simulink model "yek_alef_tanaka"  (R2024a)
settings: Solver=ode15s  StartTime=0.0  StopTime=9000  RelTol=1e-3
settings Model: Creator=MAHDI  LastModifiedBy=ASUS
settings DebuggingCC: UnconnectedInputMsg=warning  UnconnectedOutputMsg=warning  UnconnectedLineMsg=warning
settings ModelReferenceCC: EnableRefExpFcnMdlSchedulingChecks=on
settings RTWCC: GPUComputeCapability=3.5  DLArmComputeVersion=19.05

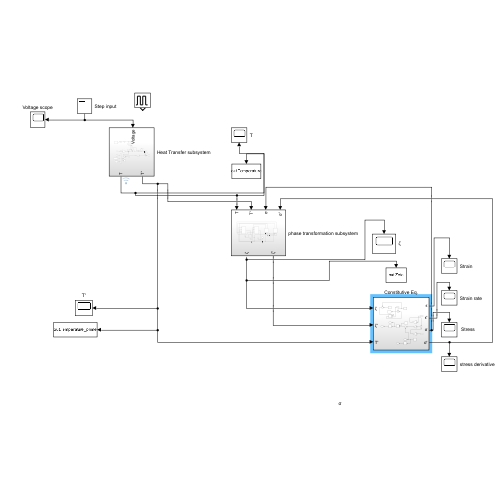
[thumbnail: Simulink's stored preview of the top-level diagram]
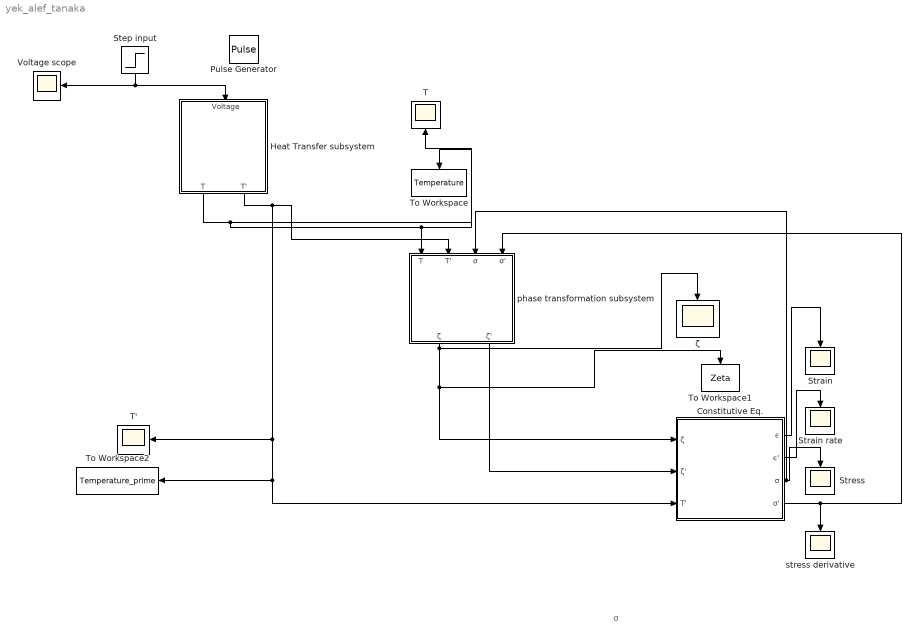
== system yek_alef_tanaka ==
  note: σ
  " Stress" : Scope
  Constitutive Eq. : Subsystem
  Heat Transfer subsystem : Subsystem
  Pulse Generator : DiscretePulseGenerator  PulseType=Time based  Period=100  PulseWidth=5
  Step input : Step  Time=70  Before=1  After=0  SampleTime=0
  Strain : Scope
  Strain rate : Scope
  T : Scope
  T' : Scope
  To Workspace : ToWorkspace  VariableName=Temperature  SampleTime=1
  To Workspace1 : ToWorkspace  VariableName=Zeta  SampleTime=1
  To Workspace2 : ToWorkspace  VariableName=Temperature_prime  SampleTime=1
  Voltage scope : Scope
  phase transformation subsystem : Subsystem
  stress derivative : Scope
  ζ : Scope
  wires:
  Constitutive Eq./3(σ) -> phase transformation subsystem/3(σ), " Stress"/1
  Step input/1 -> Voltage scope/1, Heat Transfer subsystem/1(Voltage)
  Heat Transfer subsystem/2(T') -> To Workspace2/1, Constitutive Eq./3(T'), T'/1, phase transformation subsystem/2(T')
  Heat Transfer subsystem/1(T) -> T/1, phase transformation subsystem/1(T), To Workspace/1
  phase transformation subsystem/2(ζ') -> Constitutive Eq./2(ζ')
  Constitutive Eq./1(ϵ) -> Strain/1
  phase transformation subsystem/1(ζ) -> Constitutive Eq./1(ζ), To Workspace1/1, ζ/1
  Constitutive Eq./2(ϵ') -> Strain rate/1
  Constitutive Eq./4(σ') -> phase transformation subsystem/4("σ' "), stress derivative/1

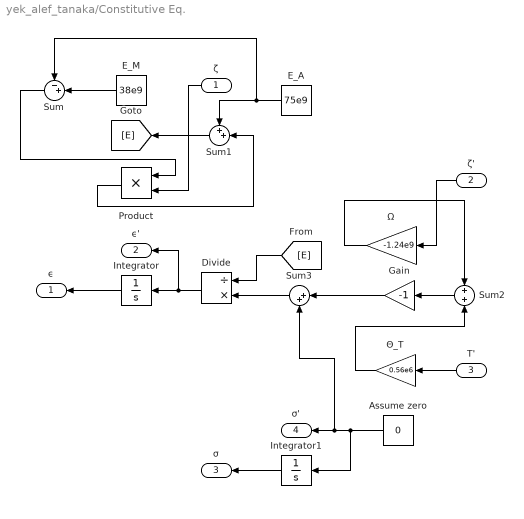
== system yek_alef_tanaka/Constitutive Eq. ==
  ζ : Inport
  ζ' : Inport  Port=2
  T' : Inport  Port=3
  Assume zero : Constant  Value=0
  Divide : Product  Inputs=/*
  E_A : Constant  Value=75e9
  E_M : Constant  Value=38e9
  Gain : Gain  Gain=-1
  Integrator : Integrator
  Integrator1 : Integrator
  Product : Product
  Sum : Sum  Inputs=-+|
  Sum1 : Sum  Inputs=++|
  Sum2 : Sum  Inputs=+|+
  Sum3 : Sum  Inputs=|++
  Θ_T : Gain  Gain=0.56e6
  Ω : Gain  Gain=-1.24e9
  ϵ : Outport
  ϵ' : Outport  Port=2
  σ : Outport  Port=3
  σ' : Outport  Port=4
  wires:
  Sum3/1 -> Divide/2
  Product/1 -> Sum1/2
  Sum1/1 -> [E]
  Sum2/1 -> Gain/1
  Integrator1/1 -> σ/1
  Sum/1 -> Product/1
  E_M/1 -> Sum/2
  E_A/1 -> Sum1/1, Sum/1
  Integrator/1 -> ϵ/1
  Divide/1 -> ϵ'/1, Integrator/1
  ζ/1 -> Product/2
  [E] -> Divide/1
  Ω/1 -> Sum2/1
  Gain/1 -> Sum3/1
  Θ_T/1 -> Sum2/2
  Assume zero/1 -> Sum3/2, σ'/1, Integrator1/1
  ζ'/1 -> Ω/1
  T'/1 -> Θ_T/1

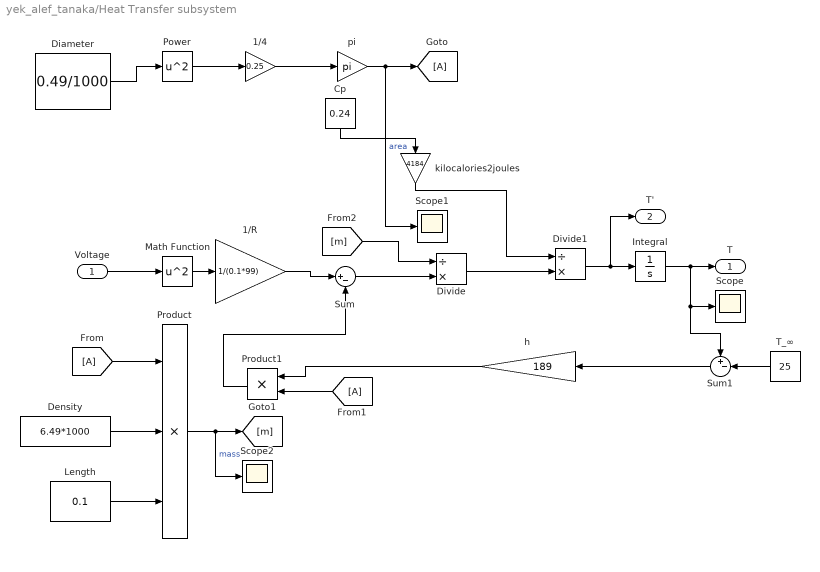
== system yek_alef_tanaka/Heat Transfer subsystem ==
  Voltage : Inport
  1/4 : Gain  Gain=0.25
  1/R : Gain  Gain=1/(0.1*99)
  Cp : Constant  Value=0.24
  Density : Constant  Value=6.49*1000
  Diameter : Constant  Value=0.49/1000
  Divide : Product  Inputs=/*
  Divide1 : Product  Inputs=/*
  From : From
  From1 : From
  Goto : Goto
  Integral : Integrator  InitialCondition=25
  Length : Constant  Value=0.1
  Math Function : Math  Operator=square
  Power : Math  Operator=square
  Product : Product  Inputs=3
  Product1 : Product
  Scope : Scope
  Scope1 : Scope
  Scope2 : Scope
  Sum : Sum  Inputs=|+-
  Sum1 : Sum  Inputs=+-|
  T_∞ : Constant  Value=25
  h : Gain  Gain=189
  "kilocalories2joules " : Gain  Gain=4184
  pi : Gain  Gain=pi
  T : Outport
  T' : Outport  Port=2
  wires:
  Voltage/1 -> Math Function/1
  Diameter/1 -> Power/1
  Density/1 -> Product/2
  From/1 -> Product/1
  1/4/1 -> pi/1
  Length/1 -> Product/3
  Product/1 -> [m], Scope2/1  "mass"
  Power/1 -> 1/4/1
  Math Function/1 -> 1/R/1
  Product1/1 -> Sum/2
  1/R/1 -> Sum/1
  Cp/1 -> "kilocalories2joules "/1
  From1/1 -> Product1/2
  pi/1 -> Scope1/1, Goto/1  "area"
  [m] -> Divide/1
  Sum/1 -> Divide/2
  "kilocalories2joules "/1 -> Divide1/1
  Divide/1 -> Divide1/2
  h/1 -> Product1/1
  Divide1/1 -> Integral/1, T'/1
  Integral/1 -> Sum1/1, Scope/1, T/1
  Sum1/1 -> h/1
  T_∞/1 -> Sum1/2

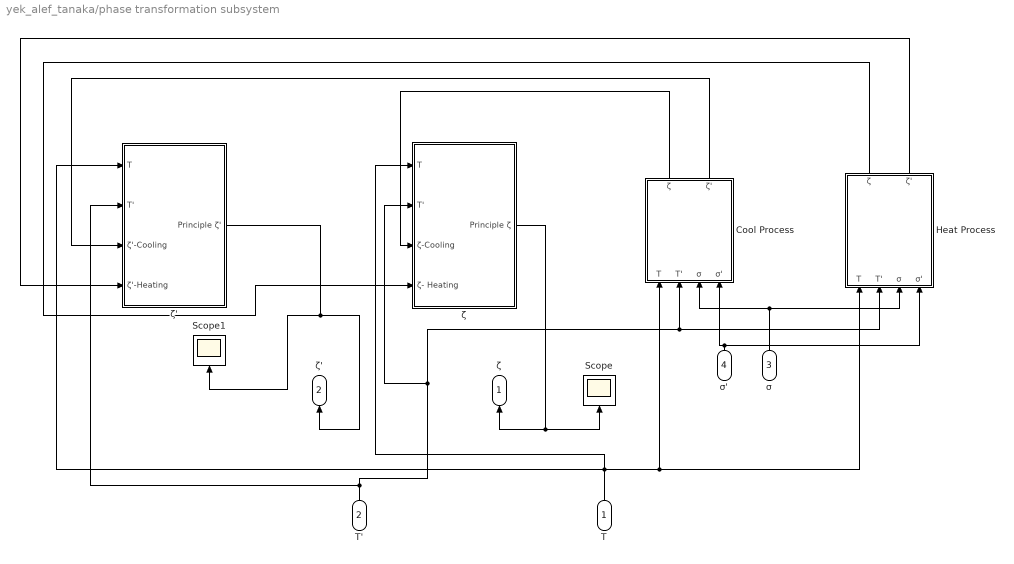
== system yek_alef_tanaka/phase transformation subsystem ==
  T : Inport
  T' : Inport  Port=2
  σ : Inport  Port=3
  "σ' " : Inport  Port=4
  " ζ" : Subsystem
  " ζ'" : Subsystem
  Cool Process : Subsystem
  Heat Process : Subsystem
  Scope : Scope
  Scope1 : Scope
  ζ : Outport
  ζ' : Outport  Port=2
  wires:
  " ζ'"/1(Principle ζ') -> ζ'/1, Scope1/1
  Heat Process/2(ζ') -> " ζ'"/4(ζ'-Heating)
  "σ' "/1 -> Heat Process/4("σ' "), Cool Process/4("σ' ")
  Heat Process/1(ζ) -> " ζ"/4(ζ- Heating)
  Cool Process/2(ζ') -> " ζ'"/3(ζ'-Cooling)
  Cool Process/1(ζ) -> " ζ"/3(ζ-Cooling)
  " ζ"/1(Principle ζ) -> ζ/1, Scope/1
  σ/1 -> Heat Process/3(σ), Cool Process/3(σ)
  T/1 -> " ζ"/1(T), Cool Process/1(T), Heat Process/1(T), " ζ'"/1(T)
  T'/1 -> Cool Process/2(T'), Heat Process/2(T'), " ζ"/2(T'), " ζ'"/2(T')

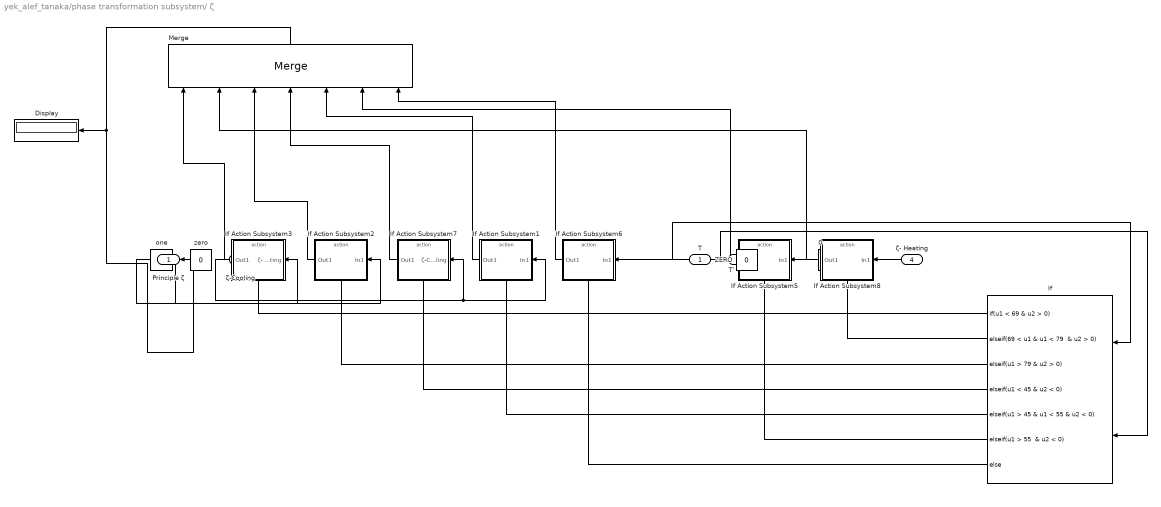
== system yek_alef_tanaka/phase transformation subsystem/ ζ ==
  T : Inport
  T' : Inport  Port=2
  ζ-Cooling : Inport  Port=3
  ζ- Heating : Inport  Port=4
  0 : Constant  Value=0
  Display : Display
  If : If  NumInputs=2  IfExpression=u1 < 69 & u2 > 0  ElseIfExpressions="69 < u1 & u1 < 79  & u2 > 0 , u1 > 79 & u2 > 0 , u1 < 45 & u2 < 0 , u1 > 45 & u1 < 55 & u2 < 0 , u1 > 55  & u2 < 0"
  If Action Subsystem1 : Subsystem  TreatAsAtomicUnit=on
  If Action Subsystem2 : Subsystem  TreatAsAtomicUnit=on
  If Action Subsystem3 : Subsystem  TreatAsAtomicUnit=on
  If Action Subsystem5 : Subsystem  TreatAsAtomicUnit=on
  If Action Subsystem6 : Subsystem  TreatAsAtomicUnit=on
  If Action Subsystem7 : Subsystem  TreatAsAtomicUnit=on
  If Action Subsystem8 : Subsystem  TreatAsAtomicUnit=on
  Merge : Merge  Inputs=7
  ZERO : Constant  Value=0
  one : Constant
  zero : Constant  Value=0
  Principle ζ : Outport
  wires:
  ζ-Cooling/1 -> If Action Subsystem7/1(ζ-Cooling), If Action Subsystem1/1(In1)
  T/1 -> If/1
  T'/1 -> If/2
  one/1 -> If Action Subsystem3/1(ζ- Heating)
  If/1 -> If Action Subsystem3/Action
  zero/1 -> If Action Subsystem2/1(In1)
  If/2 -> If Action Subsystem8/Action
  If/3 -> If Action Subsystem2/Action
  If/4 -> If Action Subsystem7/Action
  If/5 -> If Action Subsystem1/Action
  If/6 -> If Action Subsystem5/Action
  If Action Subsystem8/1(Out1) -> Merge/2
  If/7 -> If Action Subsystem6/Action
  ZERO/1 -> If Action Subsystem6/1(In1)
  0/1 -> If Action Subsystem5/1(In1)
  ζ- Heating/1 -> If Action Subsystem8/1(In1)
  If Action Subsystem3/1(Out1) -> Merge/1
  If Action Subsystem2/1(Out1) -> Merge/3
  If Action Subsystem7/1(Out1) -> Merge/4
  If Action Subsystem1/1(Out1) -> Merge/5
  If Action Subsystem6/1(Out1) -> Merge/7
  If Action Subsystem5/1(Out1) -> Merge/6
  Merge/1 -> Principle ζ/1, Display/1

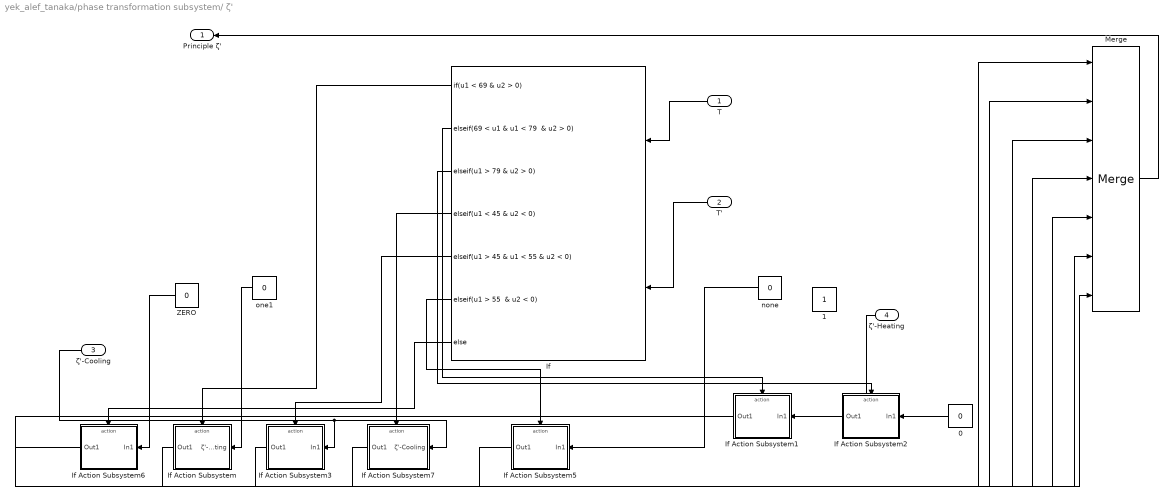
== system yek_alef_tanaka/phase transformation subsystem/ ζ' ==
  T : Inport
  T' : Inport  Port=2
  ζ'-Cooling : Inport  Port=3
  ζ'-Heating : Inport  Port=4
  0 : Constant  Value=0
  1 : Constant
  If : If  NumInputs=2  IfExpression=u1 < 69 & u2 > 0  ElseIfExpressions="69 < u1 & u1 < 79  & u2 > 0 , u1 > 79 & u2 > 0 , u1 < 45 & u2 < 0 , u1 > 45 & u1 < 55 & u2 < 0 , u1 > 55  & u2 < 0"
  If Action Subsystem : Subsystem  TreatAsAtomicUnit=on
  If Action Subsystem1 : Subsystem  TreatAsAtomicUnit=on
  If Action Subsystem2 : Subsystem  TreatAsAtomicUnit=on
  If Action Subsystem3 : Subsystem  TreatAsAtomicUnit=on
  If Action Subsystem5 : Subsystem  TreatAsAtomicUnit=on
  If Action Subsystem6 : Subsystem  TreatAsAtomicUnit=on
  If Action Subsystem7 : Subsystem  TreatAsAtomicUnit=on
  Merge : Merge  Inputs=7
  ZERO : Constant  Value=0
  none : Constant  Value=0
  one1 : Constant  Value=0
  Principle ζ' : Outport
  wires:
  If/5 -> If Action Subsystem3/Action
  ζ'-Heating/1 -> If Action Subsystem1/1(In1)
  If Action Subsystem1/1(Out1) -> Merge/2
  T'/1 -> If/2
  If Action Subsystem7/1(Out1) -> Merge/4
  If/7 -> If Action Subsystem6/Action
  0/1 -> If Action Subsystem2/1(In1)
  If Action Subsystem5/1(Out1) -> Merge/6
  T/1 -> If/1
  If/6 -> If Action Subsystem5/Action
  none/1 -> If Action Subsystem5/1(In1)
  If/4 -> If Action Subsystem7/Action
  If/3 -> If Action Subsystem2/Action
  If/2 -> If Action Subsystem1/Action
  If/1 -> If Action Subsystem/Action
  ζ'-Cooling/1 -> If Action Subsystem7/1(ζ'-Cooling), If Action Subsystem3/1(In1)
  one1/1 -> If Action Subsystem/1(ζ'-Heating)
  ZERO/1 -> If Action Subsystem6/1(In1)
  If Action Subsystem2/1(Out1) -> Merge/3
  If Action Subsystem3/1(Out1) -> Merge/5
  If Action Subsystem/1(Out1) -> Merge/1
  If Action Subsystem6/1(Out1) -> Merge/7
  Merge/1 -> Principle ζ'/1

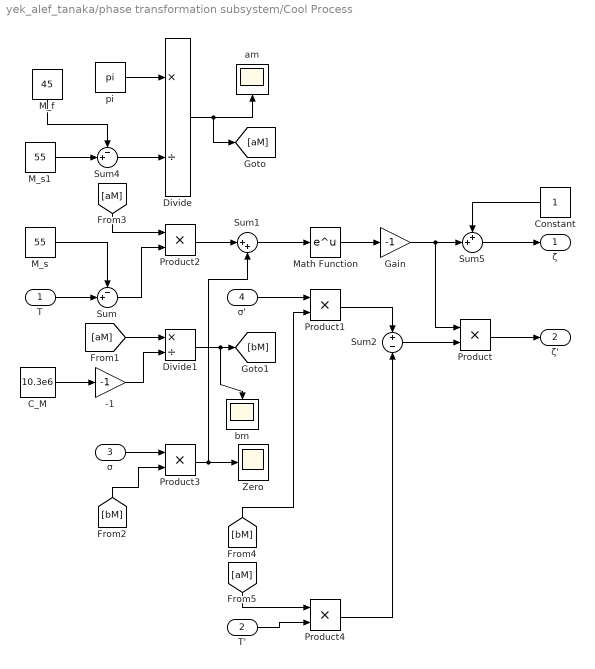
== system yek_alef_tanaka/phase transformation subsystem/Cool Process ==
  T : Inport
  T' : Inport  Port=2
  σ : Inport  Port=3
  "σ' " : Inport  Port=4
  -1 : Gain  Gain=-1
  C_M : Constant  Value=10.3e6
  Constant : Constant
  Divide : Product  Inputs=*/
  Divide1 : Product  Inputs=*/
  Gain : Gain  Gain=-1
  M_f : Constant  Value=45
  M_s : Constant  Value=55
  M_s1 : Constant  Value=55
  Math Function : Math
  Product{,1..4} (5 alike) : Product
  Sum : Sum  Inputs=-+|
  Sum1 : Sum  Inputs=|++
  Sum2 : Sum  Inputs=+|-
  Sum4 : Sum  Inputs=-+|
  Sum5 : Sum  Inputs=++|
  Zero : Scope
  am : Scope
  bm : Scope
  pi : Constant  Value=pi
  ζ : Outport
  ζ' : Outport  Port=2
  wires:
  T/1 -> Sum/2
  M_s1/1 -> Sum4/2
  M_f/1 -> Sum4/1
  M_s/1 -> Sum/1
  Product/1 -> ζ'/1
  Sum4/1 -> Divide/2
  [aM] -> Product4/1
  Product3/1 -> Sum1/2, Zero/1
  pi/1 -> Divide/1
  Product2/1 -> Sum1/1
  [aM] -> Product2/1
  Sum1/1 -> Math Function/1
  C_M/1 -> -1/1
  Sum/1 -> Product2/2
  Sum5/1 -> ζ/1
  Product1/1 -> Sum2/1
  [aM] -> Divide1/1
  -1/1 -> Divide1/2
  σ/1 -> Product3/1
  [bM] -> Product3/2
  Divide/1 -> am/1, [aM]
  Divide1/1 -> bm/1, [bM]
  "σ' "/1 -> Product1/1
  [bM] -> Product1/2
  Gain/1 -> Product/1, Sum5/2
  T'/1 -> Product4/2
  Sum2/1 -> Product/2
  Math Function/1 -> Gain/1
  Product4/1 -> Sum2/2
  Constant/1 -> Sum5/1

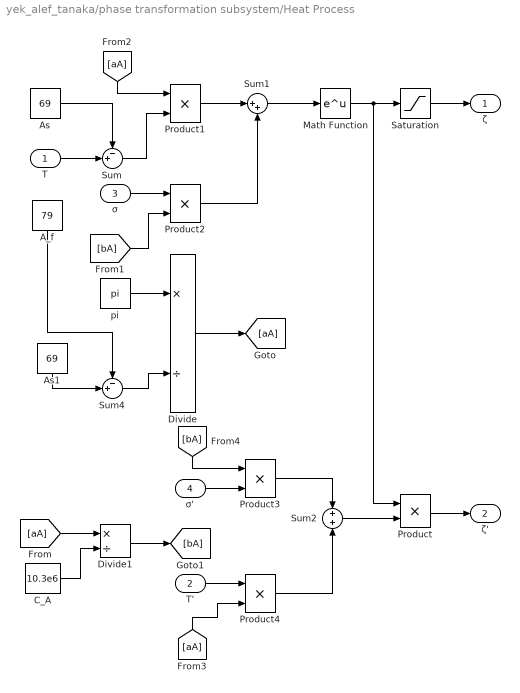
== system yek_alef_tanaka/phase transformation subsystem/Heat Process ==
  T : Inport
  T' : Inport  Port=2
  σ : Inport  Port=3
  "σ' " : Inport  Port=4
  A_f : Constant  Value=79
  As : Constant  Value=69
  As1 : Constant  Value=69
  C_A : Constant  Value=10.3e6
  Divide : Product  Inputs=*/
  Divide1 : Product  Inputs=*/
  Math Function : Math
  Product{,1..4} (5 alike) : Product
  Saturation : Saturate  UpperLimit=0.99  LowerLimit=0.01
  Sum : Sum  Inputs=-+|
  Sum1 : Sum  Inputs=|++
  Sum2 : Sum  Inputs=+|+
  Sum4 : Sum  Inputs=-+|
  pi : Constant  Value=pi
  ζ : Outport
  ζ' : Outport  Port=2
  wires:
  [aA] -> Product1/1
  [aA] -> Divide1/1
  [bA] -> Product3/1
  T/1 -> Sum/2
  As1/1 -> Sum4/2
  A_f/1 -> Sum4/1
  T'/1 -> Product4/1
  Sum/1 -> Product1/2
  Sum4/1 -> Divide/2
  C_A/1 -> Divide1/2
  Sum2/1 -> Product/2
  As/1 -> Sum/1
  σ/1 -> Product2/1
  [bA] -> Product2/2
  pi/1 -> Divide/1
  Divide1/1 -> [bA]
  Product1/1 -> Sum1/1
  Product2/1 -> Sum1/2
  Divide/1 -> [aA]
  Sum1/1 -> Math Function/1
  "σ' "/1 -> Product3/2
  Saturation/1 -> ζ/1
  [aA] -> Product4/2
  Product3/1 -> Sum2/1
  Product4/1 -> Sum2/2
  Math Function/1 -> Saturation/1, Product/1
  Product/1 -> ζ'/1

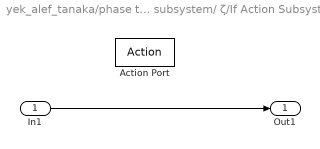
== system yek_alef_tanaka/phase transformation subsystem/ ζ/If Action Subsystem1 ==
  In1 : Inport
  Action Port : ActionPort  ActionPortLabel=elseif( u1 > 45 & u1 < 55 & u2 < 0 )
  Out1 : Outport
  wires:
  In1/1 -> Out1/1

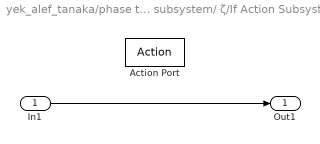
== system yek_alef_tanaka/phase transformation subsystem/ ζ/If Action Subsystem2 ==
  In1 : Inport
  Action Port : ActionPort  ActionPortLabel=elseif( u1 > 79 & u2 > 0 )
  Out1 : Outport
  wires:
  In1/1 -> Out1/1

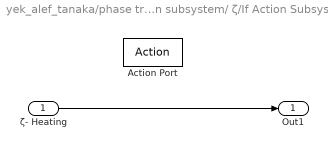
== system yek_alef_tanaka/phase transformation subsystem/ ζ/If Action Subsystem3 ==
  ζ- Heating : Inport
  Action Port : ActionPort  ActionPortLabel=if(u1 < 69 & u2 > 0)
  Out1 : Outport
  wires:
  ζ- Heating/1 -> Out1/1

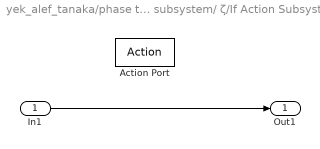
== system yek_alef_tanaka/phase transformation subsystem/ ζ/If Action Subsystem5 ==
  In1 : Inport
  Action Port : ActionPort  ActionPortLabel="elseif( u1 > 55  & u2 < 0)"
  Out1 : Outport
  wires:
  In1/1 -> Out1/1

== system yek_alef_tanaka/phase transformation subsystem/ ζ/If Action Subsystem6 ==
  In1 : Inport
  Action Port : ActionPort  ActionPortLabel=else
  Out1 : Outport
  wires:
  In1/1 -> Out1/1

== system yek_alef_tanaka/phase transformation subsystem/ ζ/If Action Subsystem7 ==
  ζ-Cooling : Inport
  Action Port : ActionPort  ActionPortLabel=elseif( u1 < 45 & u2 < 0 )
  Out1 : Outport
  wires:
  ζ-Cooling/1 -> Out1/1

== system yek_alef_tanaka/phase transformation subsystem/ ζ/If Action Subsystem8 ==
  In1 : Inport
  Action Port : ActionPort  ActionPortLabel="elseif(69 < u1 & u1 < 79  & u2 > 0 )"
  Out1 : Outport
  wires:
  In1/1 -> Out1/1

== system yek_alef_tanaka/phase transformation subsystem/ ζ'/If Action Subsystem ==
  ζ'-Heating : Inport
  Action Port : ActionPort  ActionPortLabel=if(u1 < 69 & u2 > 0)
  Out1 : Outport
  wires:
  ζ'-Heating/1 -> Out1/1

== system yek_alef_tanaka/phase transformation subsystem/ ζ'/If Action Subsystem1 ==
  In1 : Inport
  Action Port : ActionPort  ActionPortLabel="elseif(69 < u1 & u1 < 79  & u2 > 0 )"
  Out1 : Outport
  wires:
  In1/1 -> Out1/1

== system yek_alef_tanaka/phase transformation subsystem/ ζ'/If Action Subsystem2 ==
  In1 : Inport
  Action Port : ActionPort  ActionPortLabel=elseif( u1 > 79 & u2 > 0 )
  Out1 : Outport
  wires:
  In1/1 -> Out1/1

== system yek_alef_tanaka/phase transformation subsystem/ ζ'/If Action Subsystem3 ==
  In1 : Inport
  Action Port : ActionPort  ActionPortLabel=elseif( u1 > 45 & u1 < 55 & u2 < 0 )
  Out1 : Outport
  wires:
  In1/1 -> Out1/1

== system yek_alef_tanaka/phase transformation subsystem/ ζ'/If Action Subsystem5 ==
  In1 : Inport
  Action Port : ActionPort  ActionPortLabel="elseif( u1 > 55  & u2 < 0)"
  Out1 : Outport
  wires:
  In1/1 -> Out1/1

== system yek_alef_tanaka/phase transformation subsystem/ ζ'/If Action Subsystem6 ==
  In1 : Inport
  Action Port : ActionPort  ActionPortLabel=else
  Out1 : Outport
  wires:
  In1/1 -> Out1/1

== system yek_alef_tanaka/phase transformation subsystem/ ζ'/If Action Subsystem7 ==
  ζ'-Cooling : Inport
  Action Port : ActionPort  ActionPortLabel=elseif( u1 < 45 & u2 < 0 )
  Out1 : Outport
  wires:
  ζ'-Cooling/1 -> Out1/1
